simulink model "xfft"  (Simulink 7.4)
settings: Solver=ode45  StartTime=0.0  StopTime=100  RelTol=1e-3
libraries: xbsIndex_r4 x755, casper_library_misc x76, gavrt_library x8, xps_library x1, ox_lib x1
(part 1 of 9)
settings Model: Creator=jack  LastModifiedBy=jack

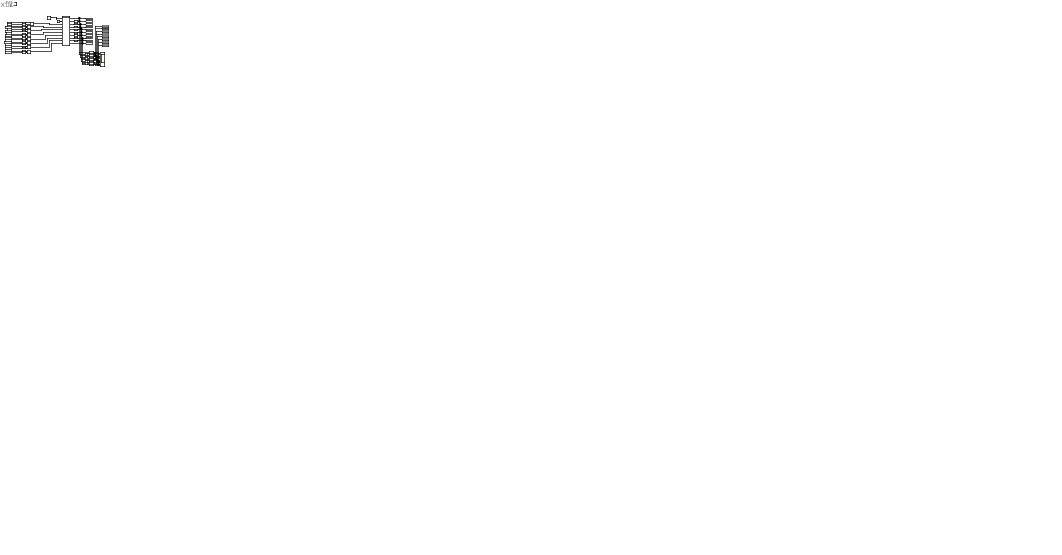
== system xfft ==
  note: what are you looking at?
  " System Generator" : xbsIndex_r4/ System Generator  Tag=genX  SystemSampleTime=-1  xilinxfamily=virtex5  part=xc5vsx95t  speed=-1  package=ff1136  synthesis_tool=XST  clock_wrapper=Clock Enables  directory=./x64_32s_001/sysgen  testbench=off  simulink_period=1  sysclk_period=4.878  dcm_input_clock_period=100  incr_netlist=off  trim_vbits=Everywhere in SubSystem  dbl_ovrd=According to Block Masks  core_generation=According to Block Masks  run_coregen=off  deprecated_control=off  eval_field=0  block_type=sysgen
      settings: block_version=11.4
  Constant1 : xbsIndex_r4/Constant  arith_type=Unsigned  const=7  n_bits=3  bin_pt=0  explicit_period=on  period=1  equ=P=C  opselect=C  inp2=PCIN>>17  opr=+  inp1=P  carry=CIN  dbl_ovrd=off  block_type=constant
      settings: block_version=11.4
  Constant{2,4..18} (16 alike) : xbsIndex_r4/Constant  arith_type=Signed (2's comp)  const=rand  n_bits=4  bin_pt=3  explicit_period=on  period=1  equ=P=C  opselect=C  inp2=PCIN>>17  opr=+  inp1=P  carry=CIN  dbl_ovrd=off  block_type=constant
      settings: block_version=11.4
  Convert{,1..15} (16 alike) : xbsIndex_r4/Convert  arith_type="Signed  (2's comp)"  n_bits=18  bin_pt=17  quantization=Truncate  overflow=Wrap  latency=0  dbl_ovrd=off  pipeline=off  block_type=convert
      settings: block_version=11.4
  Display{,1..7} (8 alike) : Display
  Gateway Out{,1..9} (10 alike) : xbsIndex_r4/Gateway Out  hdl_port=on  timing_constraint=None  locs_specified=off  LOCs={}  block_type=gatewayout
      settings: infoedit="Gateway out block.  Converts Xilinx fixed point inputs into ouputs of type Simulink integer, double, or fixed point.<br><br>Hardware notes:  In hardware these blocks become top level output ports or are discarded, depending on how they are configured."  block_version=11.4
  Scale{1..8} (8 alike) : xbsIndex_r4/Scale  scale_factor=16  dbl_ovrd=off  block_type=scale
  Scope : Scope  NumInputPorts=10
      settings: YMin=-5~-5~-5~-5~-5~-5~-5~-5~-5~-5  YMax=5~5~5~5~5~5~5~5~5~5
  XSG core config : xps_library/XSG core config  Tag=xps:xsg  SystemSampleTime=-1  hw_sys=ROACH:sx95t  ibob_linux=off  clk_src=arb_clk  iBOB_clk_src=sys_clk  BEE2_ctrl_clk_src=sys_clk  BEE2_usr_clk_src=sys_clk  ROACH_clk_src=arb_clk  CORR_clk_src=sys_clk  gpio_clk_io_group=iBOB:sma  gpio_clk_bit_index=0  clk_rate=205  sample_period=1  synthesis_tool=XST  mpc_type=powerpc440_ext
  fft_direct : Subsystem  AncestorBlock=casper_library_ffts/fft_direct  mask(fft_direct){FFTSize=3, input_bit_width=18, coeff_bit_width=18, map_tail=off, LargerFFTSize=5, StartStage=4, add_latency=1, mult_latency=2, bram_latency=2, conv_latency=1, quantization=Round  (unbiased: +/- Inf), overflow=Saturate, arch=Virtex5, opt_target=logic, coeffs_bit_limit=8, specify_mult=off, mult_spec=[2                                      2], hardcode_shifts=off, shift_schedule=[1                                      1], dsp48_adders=off}
      mask prompts: FFTSize "Size of FFT: (2^? pts)"; input_bit_width "Input/Output Bit Width"; coeff_bit_width "Coefficient Bit Width"; map_tail "Map Tail of Larger FFT"; LargerFFTSize "Size of Larger FFT (2^?)"; StartStage "Start Stage of Map Tail"; add_latency "Add Latency"; mult_latency "Mult Latency"; bram_latency "BRAM Latency"; conv_latency "Convert latency"; quantization "Quantization Behavior"; overflow "Overflow Behavior"; arch "Architecture"; opt_target "Use less"; coeffs_bit_limit "Number bits above which to store stage's coefficients in BRAM (2^? bits)"; specify_mult "Specify multiplier use (behavioural HDL if not specified)"; mult_spec "Multiplier specification (0=core, 1=behavioural HDL, 2=embedded) (left=1st stage)"; hardcode_shifts "Hardcode shift schedule"; shift_schedule "Shift schedule"; dsp48_adders "DSP48 adders in butterfly"
      mask help:
      | FFT internal block.
      |
      | Implements an N-point FFT as the classic butterfly structure,
      | with N inputs and N outputs.
      mask init:
      | fft_direct_init(gcb, ...
      |     'FFTSize', FFTSize, ...
      |     'input_bit_width', input_bit_width, ...
      |     'coeff_bit_width', coeff_bit_width, ...
      |     'map_tail', map_tail, ...
      |     'LargerFFTSize', LargerFFTSize, ...
      |     'StartStage', StartStage, ...
      |     'add_latency', add_latency, ...
      |     'mult_latency', mult_latency, ...
      |     'bram_latency', bram_latency, ...
      |     'conv_latency', conv_latency, ...
      |     'quantization', quantization, ...
      |     'overflow', overflow, ...
      |     'arch', arch, ...
      |     'opt_target', opt_target, ...
      |     'coeffs_bit_limit', coeffs_bit_limit, ...
      |     'specify_mult', specify_mult, ...
      |     'mult_spec', mult_spec, ...
      |     'hardcode_shifts', hardcode_shifts, ...
      |     'shift_schedule', shift_schedule, ...
      |     'dsp48_adders', dsp48_adders);
      settings: AttributesFormatString=|
      | Virtex5
      | stages [4  5  6] of 3
      | [18,18]
      | Round  (unbiased: +/- Inf)
      | Saturate
      mask StyleString: edit,edit,edit,checkbox,edit,edit,edit,edit,edit,edit,popup(Truncate|Round  (unbiased: +/- Inf)|Round  (unbiased: Even Values)),popup(Wrap|Saturate|Error),popup(Virtex2Pro|Virtex5),popup(logic|multipliers),edit,checkbox,edit,checkbox,edit,checkbox
      mask CallbackString:
      | |||map_tail = get_param(gcb, 'map_tail');
      | set_param_state(gcb, 'LargerFFTSize', map_tail);
      | set_param_state(gcb, 'StartStage', map_tail);|||||||||fft_callback_arch(gcb);|||specify_mult = get_param(gcb, 'specify_mult');
      | set_param_state(gcb, 'mult_spec', specify_mult);||hardcode_shifts = get_param(gcb, 'hardcode_shifts');
      | set_param_state(gcb, 'shift_schedule', hardcode_shifts);||fft_callback_dsp48_adders(gcb);
      mask TabNameString: Basic,Basic,Basic,Basic,Basic,Basic,Latency,Latency,Latency,Latency,Implementation,Implementation,Implementation,Implementation,Implementation,Implementation,Implementation,Implementation,Implementation,Implementation
  power{,1..7} (8 alike) : gavrt_library/power  SystemSampleTime=-1  BitWidth=18  add_latency=0  mult_latency=0
  ri_to_c{,1..7} (8 alike) : casper_library_misc/ri_to_c  SystemSampleTime=-1
  sim_trig : ox_lib/sim_trig  SystemSampleTime=-1  delay=10
  wires:
  fft_direct/1(sync_out) -> [x_fft_sync], Gateway Out/1
  fft_direct/10(of) -> [x_fft_of], Gateway Out9/1
  Constant1/1 -> fft_direct/2(shift)
  sim_trig/1 -> fft_direct/1(sync)
  power/1 -> [x0], Scale8/1
  power1/1 -> [x1], Scale6/1
  power2/1 -> [x2], Scale5/1
  power3/1 -> [x3], Scale4/1
  power4/1 -> [x4], Scale3/1
  power5/1 -> [x5], Scale2/1
  power6/1 -> [x6], Scale1/1
  power7/1 -> [x7], Scale7/1
  Gateway Out/1 -> Scope/1
  Gateway Out1/1 -> Scope/2, Display6/1
  Gateway Out2/1 -> Scope/3, Display7/1
  Gateway Out3/1 -> Scope/4, Display/1
  Gateway Out4/1 -> Scope/5, Display1/1
  Gateway Out5/1 -> Scope/6, Display2/1
  Gateway Out6/1 -> Scope/7, Display3/1
  Gateway Out7/1 -> Scope/8, Display4/1
  Gateway Out8/1 -> Scope/9, Display5/1
  Gateway Out9/1 -> Scope/10
  Scale8/1 -> Gateway Out1/1
  Scale6/1 -> Gateway Out2/1
  Scale5/1 -> Gateway Out3/1
  Scale4/1 -> Gateway Out4/1
  Scale3/1 -> Gateway Out5/1
  Scale2/1 -> Gateway Out6/1
  Scale1/1 -> Gateway Out7/1
  Scale7/1 -> Gateway Out8/1
  fft_direct/2(out0) -> power/1
  fft_direct/9(out7) -> power7/1
  fft_direct/3(out1) -> power1/1
  fft_direct/4(out2) -> power2/1
  fft_direct/5(out3) -> power3/1
  fft_direct/6(out4) -> power4/1
  fft_direct/7(out5) -> power5/1
  fft_direct/8(out6) -> power6/1
  Constant15/1 -> Convert1/1
  Constant13/1 -> Convert3/1
  Constant16/1 -> Convert4/1
  Constant11/1 -> Convert5/1
  Constant14/1 -> Convert6/1
  Constant10/1 -> Convert7/1
  Constant9/1 -> Convert8/1
  Constant8/1 -> Convert9/1
  Constant7/1 -> Convert10/1
  Constant6/1 -> Convert11/1
  Constant12/1 -> Convert12/1
  Constant4/1 -> Convert13/1
  Constant5/1 -> Convert14/1
  Constant2/1 -> Convert15/1
  Constant17/1 -> Convert2/1
  Constant18/1 -> Convert/1
  Convert/1 -> ri_to_c/1
  Convert1/1 -> ri_to_c/2
  Convert2/1 -> ri_to_c1/1
  Convert3/1 -> ri_to_c1/2
  Convert4/1 -> ri_to_c2/1
  Convert5/1 -> ri_to_c2/2
  Convert6/1 -> ri_to_c3/1
  Convert7/1 -> ri_to_c3/2
  Convert8/1 -> ri_to_c4/1
  Convert9/1 -> ri_to_c4/2
  Convert10/1 -> ri_to_c5/1
  Convert11/1 -> ri_to_c5/2
  Convert12/1 -> ri_to_c6/1
  Convert13/1 -> ri_to_c6/2
  Convert14/1 -> ri_to_c7/1
  Convert15/1 -> ri_to_c7/2
  ri_to_c/1 -> fft_direct/3(in0)
  ri_to_c1/1 -> fft_direct/4(in1)
  ri_to_c2/1 -> fft_direct/5(in2)
  ri_to_c3/1 -> fft_direct/6(in3)
  ri_to_c4/1 -> fft_direct/7(in4)
  ri_to_c5/1 -> fft_direct/8(in5)
  ri_to_c6/1 -> fft_direct/9(in6)
  ri_to_c7/1 -> fft_direct/10(in7)
